simulink model "LaneSimulationV1"  (R2021b)
settings: Solver=VariableStepAuto  StartTime=0.0  StopTime=10.0  RelTol=1e-3
values from neighbouring files (symbols this model uses):
  Np = 10    [acc_plot_backup.m]
  s_path = [0 1.10508939428 2.2141958029 3.32141571172 4.42705301151 5.53154548532 6.63517443471 7.73808041313 8.84055018688 9.94289959674 11.0453539299 12.1480581097 ... (1001 elements, 1001x1)]    [200_100radius.mat]    (also in LV_Clothoid_S_Turn_path.mat = [0 0.966832089581 1.93621320584 2.90214024471 3.86476766313 ; NEDC_path.mat = [0 0.414605943146 0.832514087334 1.25401518562 1.68216660344; Straight_East_into_curve.mat = [0 1.65770560069 3.32192925577 4.98420060507 6.64484613518 8; acc_plot_backup.m = Station_HV_m)
  X_path = [0 1.10508939428 2.2141958029 3.32141571172 4.42705301151 5.53154548532 6.63517443471 7.73808041313 8.84055018688 9.94289959674 11.0453539299 12.1480581097 ... (1001 elements, 1001x1)]    [200_100radius.mat]    (also in LV_Clothoid_S_Turn_path.mat = [-10 -9.03316791042 -8.06378679416 -7.09785975529 -6.1352323; NEDC_path.mat = [0 0.414605943146 0.832514087334 1.25401518562 1.68216660344; Straight_East_into_curve.mat = [0 1.65770560069 3.32192925577 4.98420060507 6.64484613518 8; acc_plot_backup.m = X_HV_m)
  Y_path = [0 -1.70364610795e-18 -7.41532896709e-18 1.46822109542e-17 4.74557362791e-17 6.12980216762e-17 9.25043977736e-17 1.24088240159e-16 1.5099156923e-16 1.7058517853e-16 1.90629227614e-16 2.09673434424e-16 ... (1001 elements, 1001x1)]    [200_100radius.mat]    (also in LV_Clothoid_S_Turn_path.mat = [0 -8.46153035536e-19 5.07382551045e-18 2.07356032218e-17 3.; NEDC_path.mat = [0 -3.50680326162e-18 -2.14111304971e-18 3.38197671014e-18 3; Straight_East_into_curve.mat = [0 1.29197709199e-18 2.81882429322e-18 3.49020462564e-17 6.7; acc_plot_backup.m = Y_HV_m)
undefined symbols (not defined in the file or in its folder): AES_pre_time, speed, t_start, Ts_MPC
(part 1 of 12)
settings Model: Creator=SheonSu  LastModifiedBy=SheonSu

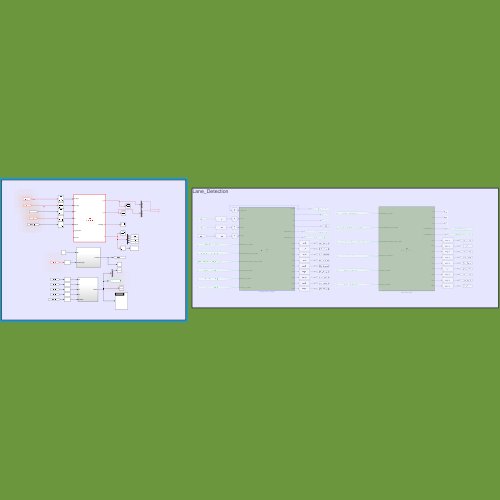
[thumbnail: Simulink's stored preview of the top-level diagram]
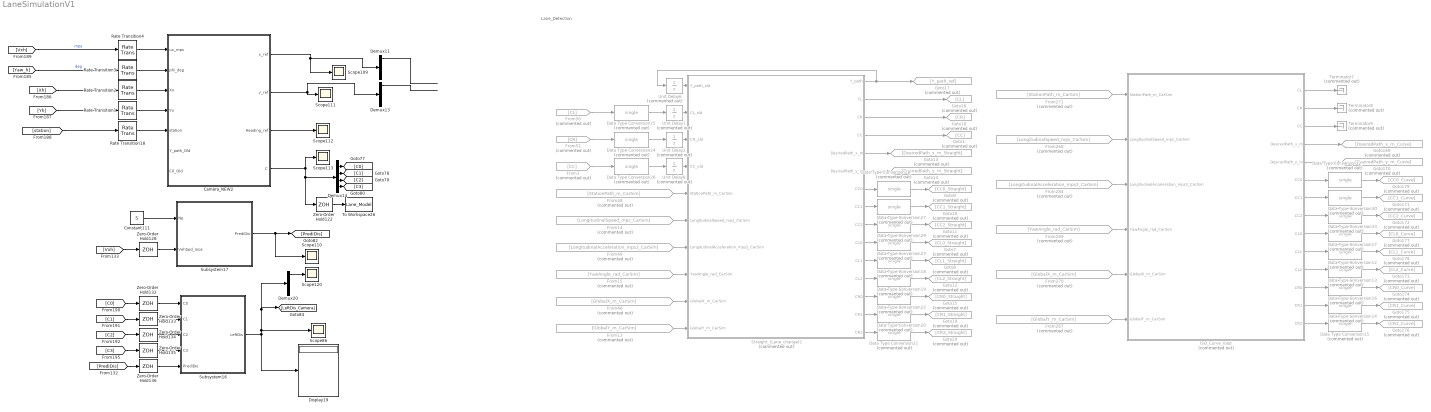
== system LaneSimulationV1 ==
  note: Lane_Detection
  Camera_NEW2 : MATLAB Function  TreatAsAtomicUnit=on
  Constant111 : Constant  Value=5
  Data Type Conversion{12..30,32..33} (21 alike) : DataTypeConversion  Commented=on  OutDataTypeStr=single
  Demux11 : Demux  Outputs=5
  Demux13 : Demux  Outputs=5
  Demux14 : Demux
  Demux20 : Demux  Outputs=5
  Display19 : Display
  From1 : From  Commented=on  GotoTag=CC
  From13 : From  Commented=on  GotoTag=GlobalY_m_CarSim
  From14 : From  Commented=on  GotoTag=LongitudinalSpeed_mps_CarSim
  From15 : From  Commented=on  GotoTag=YawAngle_rad_CarSim
  From267 : From  Commented=on  GotoTag=GlobalY_m_CarSim
  From268 : From  Commented=on  GotoTag=LongitudinalSpeed_mps_CarSim
  From269 : From  Commented=on  GotoTag=YawAngle_rad_CarSim
  From270 : From  Commented=on  GotoTag=GlobalX_m_CarSim
  From271 : From  Commented=on  GotoTag=StationPath_m_CarSim
  From284 : From  Commented=on  GotoTag=LongitudinalAcceleration_mps2_CarSim
  From46 : From  Commented=on  GotoTag=GlobalX_m_CarSim
  From48 : From  Commented=on  GotoTag=StationPath_m_CarSim
  From49 : From  Commented=on  GotoTag=LongitudinalAcceleration_mps2_CarSim
  From50 : From  Commented=on  GotoTag=CL
  From51 : From  Commented=on  GotoTag=CR
  Goto1 : Goto  Commented=on  GotoTag=CC
  Goto10 : Goto  Commented=on  GotoTag=CC1_Straight
  Goto11 : Goto  Commented=on  GotoTag=CC2_Straight
  Goto12 : Goto  Commented=on  GotoTag=CL2_Straight
  Goto13 : Goto  Commented=on  GotoTag=DseiredPath_x_m_Straight
  Goto14 : Goto  Commented=on  GotoTag=DseiredPath_y_m_Straight
  Goto15 : Goto  Commented=on  GotoTag=CR0_Straight
  Goto16 : Goto  Commented=on  GotoTag=CL
  Goto169 : Goto  Commented=on  GotoTag=DseiredPath_x_m_Curve
  Goto17 : Goto  Commented=on  GotoTag=Y_path_ref
  Goto170 : Goto  Commented=on  GotoTag=DseiredPath_y_m_Curve
  Goto171 : Goto  Commented=on  GotoTag=CC1_Curve
  Goto172 : Goto  Commented=on  GotoTag=CC2_Curve
  Goto173 : Goto  Commented=on  GotoTag=CL2_Curve
  Goto174 : Goto  Commented=on  GotoTag=CR0_Curve
  Goto175 : Goto  Commented=on  GotoTag=CR1_Curve
  Goto176 : Goto  Commented=on  GotoTag=CR2_Curve
  Goto177 : Goto  Commented=on  GotoTag=CL0_Curve
  Goto178 : Goto  Commented=on  GotoTag=CL1_Curve
  Goto179 : Goto  Commented=on  GotoTag=CC0_Curve
  Goto18 : Goto  Commented=on  GotoTag=CR
  Goto19 : Goto  Commented=on  GotoTag=CR1_Straight
  Goto20 : Goto  Commented=on  GotoTag=CR2_Straight
  Goto7 : Goto  Commented=on  GotoTag=CL0_Straight
  Goto8 : Goto  Commented=on  GotoTag=CL1_Straight
  Goto9 : Goto  Commented=on  GotoTag=CC0_Straight
  ISO_Curve_road : MATLAB Function  Commented=on  TreatAsAtomicUnit=on
  Rate Transition{1..4,18} (5 alike) : RateTransition  OutPortSampleTime=0.1
  Scope{86,109..113,120} (7 alike) : Scope
  Straight_(Lane_change)1 : MATLAB Function  Commented=on  TreatAsAtomicUnit=on
  Subsystem16 : Subsystem
  Subsystem17 : Subsystem
  Terminator7 : Terminator  Commented=on
  Terminator8 : Terminator  Commented=on
  Terminator9 : Terminator  Commented=on
  To Workspace26 : ToWorkspace  VariableName=Lane_Model  SampleTime=-1
  Unit Delay1 : UnitDelay  Commented=on  InitialCondition=[0 0 1.75]  SampleTime=-1  HasFrameUpgradeWarning=on
  Unit Delay2 : UnitDelay  Commented=on  InitialCondition=[0 0 -1.75]  SampleTime=-1  HasFrameUpgradeWarning=on
  Unit Delay6 : UnitDelay  Commented=on  InitialCondition=[0 0 0 0]  SampleTime=-1  HasFrameUpgradeWarning=on
  Unit Delay8 : UnitDelay  Commented=on  InitialCondition=[0 0 1.75]  SampleTime=-1  HasFrameUpgradeWarning=on
  Zero-Order Hold122 : ZeroOrderHold  SampleTime=0.0005
  Zero-Order Hold{128,132..136} (6 alike) : ZeroOrderHold  SampleTime=0.1
  wires:
  [Vxh] -> Zero-Order Hold128/1
  Zero-Order Hold132/1 -> Subsystem16/1(C0)
  Demux14/4 -> [C3]
  Demux14/2 -> [C1]
  Camera_NEW2/4(C) -> Zero-Order Hold122/1, Demux14/1, Scope113/1
  Zero-Order Hold128/1 -> Subsystem17/2(VehSpd_mps)
  Camera_NEW2/2(y_ref) -> Demux13/1, Scope111/1
  Constant111/1 -> Subsystem17/1(Np)
  Camera_NEW2/1(x_ref) -> Scope109/1, Demux11/1
  [C1] -> Zero-Order Hold133/1
  Demux11/1 -> ?
  Subsystem16/1(LeftDis) -> Display19/1, Demux20/1, [LeftDis_Camera], Scope86/1
  Demux13/1 -> ?
  Zero-Order Hold122/1 -> To Workspace26/1
  [Vxh] -> Rate Transition4/1  "mps"
  Demux20/1 -> Scope120/1
  Zero-Order Hold136/1 -> Subsystem16/5(PrediDis)
  Subsystem17/1(PrediDis) -> Scope110/1, [PrediDis]
  Zero-Order Hold135/1 -> Subsystem16/4(C3)
  Zero-Order Hold133/1 -> Subsystem16/2(C1)
  Demux14/1 -> [C0]
  Rate Transition4/1 -> Camera_NEW2/1(ux_mps)
  [C0] -> Zero-Order Hold132/1
  Camera_NEW2/3(Heading_ref) -> Scope112/1
  [C3] -> Zero-Order Hold135/1
  [C2] -> Zero-Order Hold134/1
  Zero-Order Hold134/1 -> Subsystem16/3("C2 ")
  Rate Transition18/1 -> Camera_NEW2/5(station)
  Rate Transition2/1 -> Camera_NEW2/3(Xo)
  [station] -> Rate Transition18/1
  [Yaw_h] -> Rate Transition3/1  "deg"
  [Xh] -> Rate Transition2/1
  [Yh] -> Rate Transition1/1
  [PrediDis] -> Zero-Order Hold136/1
  Rate Transition3/1 -> Camera_NEW2/2(phi_deg)
  Demux14/3 -> [C2]
  Rate Transition1/1 -> Camera_NEW2/4(Yo)
  Data Type Conversion25/1 -> Unit Delay1/1
  ISO_Curve_road/7(CC1) -> Data Type Conversion30/1
  From284/1 -> ISO_Curve_road/3(LongitudinalAcceleration_mps2_CarSim)
  From15/1 -> Straight_(Lane_change)1/8(YawAngle_rad_CarSim)
  ISO_Curve_road/12(CR0) -> Data Type Conversion16/1
  Data Type Conversion20/1 -> Goto19/1
  Straight_(Lane_change)1/10(CL0) -> Data Type Conversion23/1
  Straight_(Lane_change)1/9(CC2) -> Data Type Conversion29/1
  ISO_Curve_road/14(CR2) -> Data Type Conversion15/1
  Unit Delay6/1 -> Straight_(Lane_change)1/1(Y_path_old)
  Data Type Conversion15/1 -> Goto176/1
  Straight_(Lane_change)1/4(CC) -> Goto1/1
  Straight_(Lane_change)1/13(CR0) -> Data Type Conversion22/1
  Data Type Conversion14/1 -> Goto175/1
  Data Type Conversion19/1 -> Goto12/1
  Data Type Conversion13/1 -> Goto173/1
  Data Type Conversion26/1 -> Unit Delay8/1
  Straight_(Lane_change)1/3(CR) -> Goto18/1
  From1/1 -> Data Type Conversion26/1
  Unit Delay8/1 -> Straight_(Lane_change)1/4(CC_old)
  Data Type Conversion24/1 -> Unit Delay2/1
  From268/1 -> ISO_Curve_road/2(LongitudinalSpeed_mps_CarSim)
  Data Type Conversion21/1 -> Goto20/1
  From269/1 -> ISO_Curve_road/4(YawAngle_rad_CarSim)
  ISO_Curve_road/5(DesiredPath_y_m) -> Goto170/1
  From267/1 -> ISO_Curve_road/6(GlobalY_m_CarSim)
  From49/1 -> Straight_(Lane_change)1/7(LongitudinalAcceleration_mps2_CarSim)
  ISO_Curve_road/9(CL0) -> Data Type Conversion17/1
  ISO_Curve_road/8(CC2) -> Data Type Conversion33/1
  Data Type Conversion33/1 -> Goto172/1
  Data Type Conversion16/1 -> Goto174/1
  ISO_Curve_road/10(CL1) -> Data Type Conversion12/1
  ISO_Curve_road/2(CR) -> Terminator8/1
  Straight_(Lane_change)1/11(CL1) -> Data Type Conversion18/1
  Data Type Conversion23/1 -> Goto7/1
  Data Type Conversion27/1 -> Goto10/1
  ISO_Curve_road/3(CC) -> Terminator9/1
  Straight_(Lane_change)1/6(DesiredPath_y_m) -> Goto14/1
  From51/1 -> Data Type Conversion24/1
  Straight_(Lane_change)1/15(CR2) -> Data Type Conversion21/1
  Unit Delay2/1 -> Straight_(Lane_change)1/3(CR_old)
  Data Type Conversion32/1 -> Goto179/1
  From270/1 -> ISO_Curve_road/5(GlobalX_m_CarSim)
  From13/1 -> Straight_(Lane_change)1/10(GlobalY_m_CarSim)
  ISO_Curve_road/11(CL2) -> Data Type Conversion13/1
  ISO_Curve_road/6(CC0) -> Data Type Conversion32/1
  Data Type Conversion12/1 -> Goto178/1
  Straight_(Lane_change)1/8(CC1) -> Data Type Conversion27/1
  Unit Delay1/1 -> Straight_(Lane_change)1/2(CL_old)
  Straight_(Lane_change)1/1(Y_path) -> Unit Delay6/1, Goto17/1
  From46/1 -> Straight_(Lane_change)1/9(GlobalX_m_CarSim)
  Straight_(Lane_change)1/2(CL) -> Goto16/1
  Data Type Conversion29/1 -> Goto11/1
  From271/1 -> ISO_Curve_road/1(StationPath_m_CarSim)
  From50/1 -> Data Type Conversion25/1
  Straight_(Lane_change)1/5(DesiredPath_x_m) -> Goto13/1
  Straight_(Lane_change)1/7(CC0) -> Data Type Conversion28/1
  From48/1 -> Straight_(Lane_change)1/5(StationPath_m_CarSim)
  Data Type Conversion30/1 -> Goto171/1
  Straight_(Lane_change)1/12(CL2) -> Data Type Conversion19/1
  Data Type Conversion17/1 -> Goto177/1
  ISO_Curve_road/13(CR1) -> Data Type Conversion14/1
  Data Type Conversion22/1 -> Goto15/1
  Data Type Conversion28/1 -> Goto9/1
  ISO_Curve_road/4(DesiredPath_x_m) -> Goto169/1
  ISO_Curve_road/1(CL) -> Terminator7/1
  From14/1 -> Straight_(Lane_change)1/6(LongitudinalSpeed_mps_CarSim)
  Data Type Conversion18/1 -> Goto8/1
  Straight_(Lane_change)1/14(CR1) -> Data Type Conversion20/1

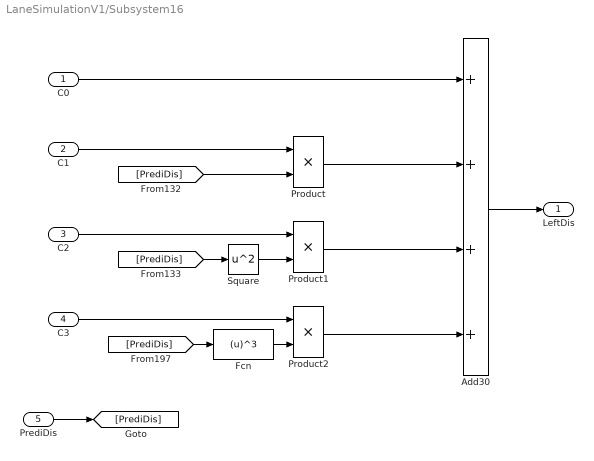
== system LaneSimulationV1/Subsystem16 ==
  C0 : Inport
  C1 : Inport  Port=2
  "C2 " : Inport  Port=3
  C3 : Inport  Port=4
  PrediDis : Inport  Port=5
  Add30 : Sum  Inputs=++++
  Fcn : Fcn  Expr=(u)^3
  Product : Product
  Product1 : Product
  Product2 : Product
  Square : Math  Operator=square  SignedPower=on  RndMeth=Zero  SaturateOnIntegerOverflow=on
  LeftDis : Outport  VectorParamsAs1DForOutWhenUnconnected=off
  wires:
  C3/1 -> Product2/1
  Add30/1 -> LeftDis/1
  C1/1 -> Product/1
  Product2/1 -> Add30/4
  C0/1 -> Add30/1
  Square/1 -> Product1/2
  Fcn/1 -> Product2/2
  [PrediDis] -> Fcn/1
  [PrediDis] -> Product/2
  "C2 "/1 -> Product1/1
  Product1/1 -> Add30/3
  Product/1 -> Add30/2
  [PrediDis] -> Square/1
  PrediDis/1 -> [PrediDis]

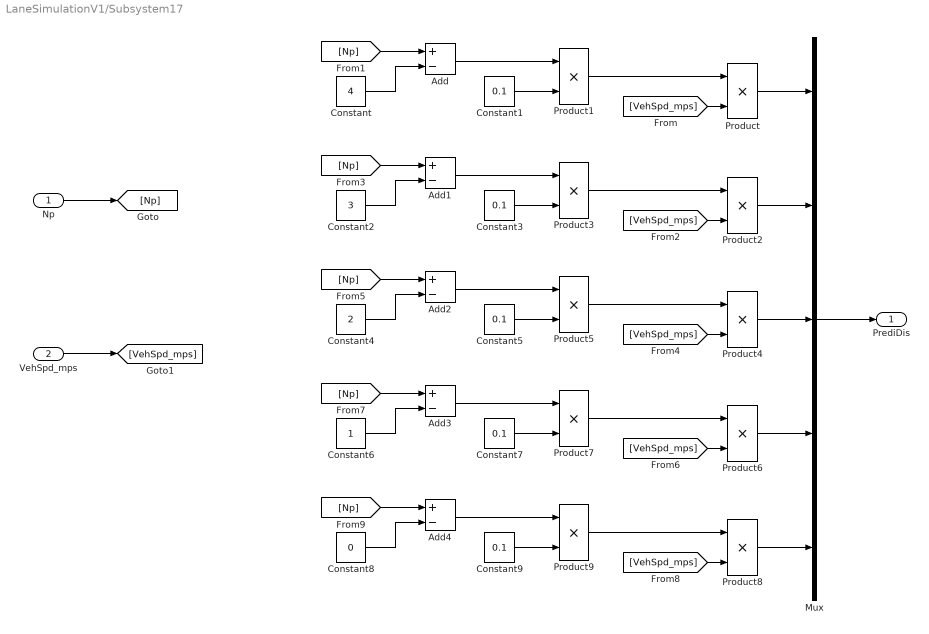
== system LaneSimulationV1/Subsystem17 ==
  Np : Inport
  VehSpd_mps : Inport  Port=2
  Add{,1..4} (5 alike) : Sum  Inputs=+-
  Constant : Constant  Value=4
  Constant{1,3,5,7,9} (5 alike) : Constant  Value=0.1
  Constant2 : Constant  Value=3
  Constant4 : Constant  Value=2
  Constant6 : Constant
  Constant8 : Constant  Value=0
  Mux : Mux  Inputs=5
  Product{,1..9} (10 alike) : Product
  PrediDis : Outport  VectorParamsAs1DForOutWhenUnconnected=off
  wires:
  Mux/1 -> PrediDis/1
  Np/1 -> [Np]
  VehSpd_mps/1 -> [VehSpd_mps]
  Product/1 -> Mux/1
  [VehSpd_mps] -> Product/2
  Product1/1 -> Product/1
  Add/1 -> Product1/1
  [Np] -> Add/1
  Constant/1 -> Add/2
  Constant1/1 -> Product1/2
  Constant3/1 -> Product3/2
  Constant2/1 -> Add1/2
  [Np] -> Add1/1
  Add1/1 -> Product3/1
  Product3/1 -> Product2/1
  [VehSpd_mps] -> Product2/2
  Product2/1 -> Mux/2
  [VehSpd_mps] -> Product4/2
  Product5/1 -> Product4/1
  Add2/1 -> Product5/1
  [Np] -> Add2/1
  Constant4/1 -> Add2/2
  Constant5/1 -> Product5/2
  Product4/1 -> Mux/3
  Product6/1 -> Mux/4
  Constant7/1 -> Product7/2
  Constant6/1 -> Add3/2
  [Np] -> Add3/1
  Add3/1 -> Product7/1
  Product7/1 -> Product6/1
  [VehSpd_mps] -> Product6/2
  [VehSpd_mps] -> Product8/2
  Product9/1 -> Product8/1
  Add4/1 -> Product9/1
  [Np] -> Add4/1
  Constant8/1 -> Add4/2
  Constant9/1 -> Product9/2
  Product8/1 -> Mux/5
